simulink model "singlePhaseMMCfaultSimplev4"  (R2023b)
settings: Solver=FixedStepDiscrete  StartTime=0.0  StopTime=20  RelTol=1e-3
PreLoadFcn:
  | % Nominal system frequency (Hz)
  |     Fnom= 50;
  | % Number of power module per half-arm
  |     Nb_PM=4;
  | % Nominal DC voltage of one module (V)
  |     Vnom_PM=1000;
  | % Nominal voltage plus DC source
  |     VDCp= (Nb_PM*Vnom_PM)/2;
  | % Nominal voltage minus DC source
  |     VDCm= VDCp;
  | % Power module capacitor (F)
  |     C_PM= 1e9;
  | % Initial capacitor DC voltage (V)
  |     Vc_Initial=Vnom_PM;
  | % SPS Simulation time step(s)
  |     Ts_Power= 10e-6;
  | 
  | % Modulator Parameters:
  | % Carriers frequency (Hz)
  |     Fc=Fnom*3;
  | 
  | % Switches parameters:
  | Ron=1e-3;
  | Rs=1e6;
  | Cs=inf;
libraries: spsHalfBridgeMMCLib x8, spsSeriesRLCBranchLib x6, spsIdealSwitchLib x4, spsVoltageMeasurementLib x4, spsCurrentMeasurementLib x3, spsPWMGeneratorMultilevelLib x2, spsGroundLib x2, spsDCVoltageSourceLib x2, spspowerguiLib x1
settings Model: Creator=The MathWorks, Inc.  LastModifiedBy=broom
settings SolverCC: AlgebraicLoopSolver=TrustRegion
settings DataIOCC: SaveFormat=StructureWithTime  SaveOutput=off  SignalLogging=off  DSMLogging=off  SaveTime=off  ReturnWorkspaceOutputs=off
settings OptimizationCC: ExpressionDepthLimit=2147483647  LifeSpan=inf
settings DebuggingCC: UnderspecifiedInitializationDetection=Classic  MergeDetectMultiDrivingBlocksExec=none  SolverPrmCheckMsg=warning  FcnCallInpInsideContextMsg=warning  UnconnectedInputMsg=warning  UnconnectedOutputMsg=warning  UnconnectedLineMsg=warning  AllowSymbolicDim=off  StateNameClashWarn=warning  SFUnexpectedBacktrackingDiag=warning  SFNoUnconditionalDefaultTransitionDiag=warning  SFExecutionAtInitializationDiag=none  ArithmeticOperatorsInVariantConditions=warning
settings HardwareCC: ProdBitPerPointer=32  ProdBitPerSizeT=32  ProdBitPerPtrDiffT=32  ProdLargestAtomicFloat=None  ProdIntDivRoundTo=Undefined  ProdEndianess=Unspecified  ProdWordSize=32  ProdHWDeviceType=32-bit Generic
settings ModelReferenceCC: EnableRefExpFcnMdlSchedulingChecks=on  PropagateSignalLabelsOutOfModel=off
settings SFSimCC: SimUseLocalCustomCode=off  CustomCodeUndefinedFunction=UseInterfaceOnly
settings RTWCC: RTWUseLocalCustomCode=off
settings CodeAppCC: StateflowObjectComments=on
settings GRTTargetCC: TargetLangStandard=C89/C90 (ANSI)  CombineOutputUpdateFcns=off  GRTInterface=on
settings ConfigComp: CovMetricSettings=dw  CovSaveCumulativeToWorkspaceVar=on  CovSaveSingleToWorkspaceVar=on  CovExternalEMLEnable=off
settings SimscapeCC: SimscapeNormalizeSystem=off  SimscapeNominalValues={1, 'bar'; 1, 'cm^3/s'; 1, 'bar*kg/s'; 1, 'kJ/kg'; 1, 'kW'; }

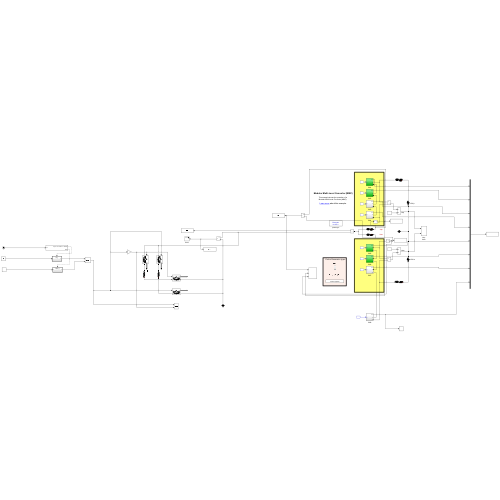
[thumbnail: Simulink's stored preview of the top-level diagram]
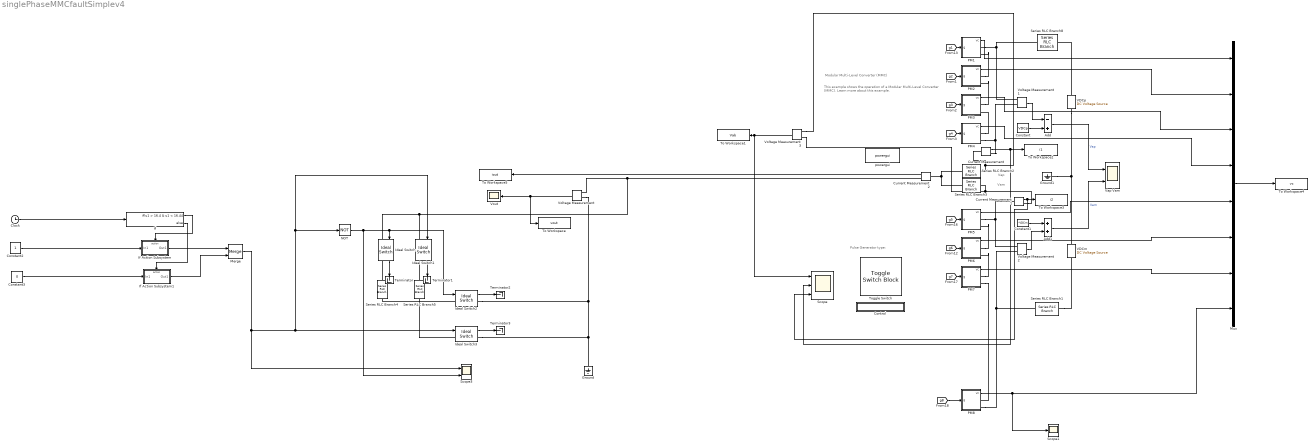
== system singlePhaseMMCfaultSimplev4 ==
  note: Pulse Generator type:
  note: Vap
  note: Vam
  note: Modular Multi-Level Converter (MMC)
  note: This example shows the operation of a
      | Modular Multi-Level Converter (MMC).
      |
      | Learn more about this example.
  Add : Sum  Inputs=-+
  Add1 : Sum
  Clock : Clock
  Constant : Constant  Value=VDCp
  Constant1 : Constant  Value=-VDCm
  Constant2 : Constant
  Constant3 : Constant  Value=0
  Control : Subsystem
      mask Display: disp('Control system')
  Current Measurement : spsCurrentMeasurementLib/Current Measurement  PhasorSimulation=off  OutputType=Complex  PSBequivalent=0
  Current Measurement1 : spsCurrentMeasurementLib/Current Measurement  PhasorSimulation=off  OutputType=Complex  PSBequivalent=0
  Current Measurement2 : spsCurrentMeasurementLib/Current Measurement  PhasorSimulation=off  OutputType=Complex  PSBequivalent=0
  Ground : spsGroundLib/Ground  LConnTagsString=a
  Ground1 : spsGroundLib/Ground  LConnTagsString=a
  Ideal Switch : spsIdealSwitchLib/Ideal Switch  Ron=0.001  Lon=0  IC=1  Rs=1e5  Cs=inf  Measurements=on
  Ideal Switch1 : spsIdealSwitchLib/Ideal Switch  Ron=0.001  Lon=0  IC=0  Rs=1e5  Cs=inf  Measurements=on
  Ideal Switch2 : spsIdealSwitchLib/Ideal Switch  Ron=0.001  Lon=0  IC=1  Rs=1e5  Cs=inf  Measurements=on
  Ideal Switch3 : spsIdealSwitchLib/Ideal Switch  Ron=0.001  Lon=0  IC=0  Rs=1e5  Cs=inf  Measurements=on
  If : If  IfExpression=u1 > 16.4 & u1 < 16.44
  If Action Subsystem : Subsystem  TreatAsAtomicUnit=on
  If Action Subsystem1 : Subsystem  TreatAsAtomicUnit=on
  Merge : Merge
  Mux : Mux  Inputs=8
  NOT : Logic  Operator=NOT  IconShape=distinctive  AllPortsSameDT=off  OutDataTypeStr=boolean
  PM1 : Subsystem
  PM2 : Subsystem
  PM3 : Subsystem
  PM4 : Subsystem
  PM5 : Subsystem
  PM6 : Subsystem
  PM7 : Subsystem
  PM8 : Subsystem
  Scope : Scope  NumInputPorts=3
  Scope1 : Scope
  Scope3 : Scope  NumInputPorts=2
  Series RLC Branch1 : spsSeriesRLCBranchLib/Series RLC Branch  LConnTagsString=__new0  RConnTagsString=__new0  BranchType=RL  Resistance=0.1  Inductance=1e-3  SetiL0=off  InitialCurrent=0  Capacitance=1e-6  Setx0=off  InitialVoltage=0  Measurements=None
  Series RLC Branch2 : spsSeriesRLCBranchLib/Series RLC Branch  LConnTagsString=__new0  RConnTagsString=__new0  BranchType=RL  Resistance=1  Inductance=10e-3  SetiL0=off  InitialCurrent=0  Capacitance=1e-6  Setx0=off  InitialVoltage=0  Measurements=None
  Series RLC Branch3 : spsSeriesRLCBranchLib/Series RLC Branch  LConnTagsString=__new0  RConnTagsString=__new0  BranchType=RL  Resistance=1  Inductance=10e-3  SetiL0=off  InitialCurrent=0  Capacitance=1e-6  Setx0=off  InitialVoltage=0  Measurements=None
  Series RLC Branch4 : spsSeriesRLCBranchLib/Series RLC Branch  LConnTagsString=__new0  RConnTagsString=__new0  BranchType=R  Resistance=50  Inductance=10e-3  SetiL0=off  InitialCurrent=0  Capacitance=1e-6  Setx0=off  InitialVoltage=0  Measurements=None
  Series RLC Branch5 : spsSeriesRLCBranchLib/Series RLC Branch  LConnTagsString=__new0  RConnTagsString=__new0  BranchType=R  Resistance=1e-9  Inductance=10e-3  SetiL0=off  InitialCurrent=0  Capacitance=1e-6  Setx0=off  InitialVoltage=0  Measurements=None
  Series RLC Branch8 : spsSeriesRLCBranchLib/Series RLC Branch  LConnTagsString=__new0  RConnTagsString=__new0  BranchType=RL  Resistance=0.1  Inductance=1e-3  SetiL0=off  InitialCurrent=0  Capacitance=1e-6  Setx0=off  InitialVoltage=0  Measurements=None
  Terminator{,1..3} (4 alike) : Terminator
  To Workspace : ToWorkspace  VariableName=vout  SaveFormat=Timeseries  SampleTime=-1
  To Workspace1 : ToWorkspace  VariableName=Vab  SaveFormat=Timeseries  SampleTime=-1
  To Workspace2 : ToWorkspace  VariableName=i1  SaveFormat=Timeseries  SampleTime=-1
  To Workspace3 : ToWorkspace  VariableName=i2  SaveFormat=Timeseries  SampleTime=-1
  To Workspace4 : ToWorkspace  VariableName=vc  SaveFormat=Timeseries  SampleTime=-1
      settings: Save2DSignal=2-D array (concatenate along first dimension)
  To Workspace5 : ToWorkspace  VariableName=iout  SaveFormat=Timeseries  SampleTime=-1
  Toggle Switch : ToggleSwitchBlock  LabelPosition=Hide
      settings: Values={{'Nearest level', 'PWM'}, [0 1]}
  VDCm : spsDCVoltageSourceLib/DC Voltage Source  Amplitude=VDCm  Measurements=None
  VDCp : spsDCVoltageSourceLib/DC Voltage Source  Amplitude=VDCp  Measurements=None
  Vap Vam : Scope  NumInputPorts=2
  Voltage Measurement{,1..3} (4 alike) : spsVoltageMeasurementLib/Voltage Measurement  PhasorSimulation=off  OutputType=Complex  PSBequivalent=0
  Vout : Scope
  powergui : spspowerguiLib/powergui  Priority=1  SimulationMode=Discrete  SampleTime=Ts_Power  frequency=60  Iterations=50  frequencyindice=0  Pbase=100e6  ErrMax=1e-4  UnitsV=kV  UnitsW=MW  buscounter=0  FunctionMessages=off  echomessages=off  EnableUseOfTLC=off  CurrentSourceSwitches=off  DisableSnubberDevices=off  DisableRonSwitches=off  DisableVfSwitches=off  DisplayEquations=off  AutomaticDiscreteSolvers=off  SolverType=Tustin/Backward Euler (TBE)  Interpol=off  ExternalGateDelay=off  methode=off  Ts=10  x0status=blocks  SPID=off  SwTol=0  HookPort=off  NonlinearTolerance=1e-4  nMaxIteration=100  ContinueOnMaxIteration=off  RestoreLinks=warning  ResistiveCurrentMeasurement=off  Frange=[0:2:500]  Ylog=off  Xlog=on  ShowGrid=off  save=off  variable=ZData  structure=Vout  ZoomFFT=on  StartTime=0.15  cycles=2  DisplayStyle=1  fundamental=50  FreqAxis=on  MaxFrequency=6000  frequencyindicesteady=1  RmsSteady=1  display=off
  wires:
  [g1] -> PM1/1(g)
  [g2] -> PM2/1(g)
  [g3] -> PM3/1(g)
  [g4] -> PM4/1(g)
  [g5] -> PM5/1(g)
  [g6] -> PM6/1(g)
  [g7] -> PM7/1(g)
  Voltage Measurement/1 -> To Workspace/1, Vout/1
  Voltage Measurement1/1 -> Add/1
  Add/1 -> Vap Vam/1  "Vap"
  Add1/1 -> Vap Vam/2  "Vam"
  Constant/1 -> Add/2
  Constant1/1 -> Add1/1
  Voltage Measurement2/1 -> Add1/2
  Voltage Measurement3/1 -> Scope/1, To Workspace1/1
  Current Measurement/1 -> To Workspace2/1, Scope/2
  Current Measurement1/1 -> Scope/3, To Workspace3/1
  PM1/1(vc) -> Mux/1
  PM2/1(vc) -> Mux/2
  PM3/1(vc) -> Mux/3
  PM4/1(vc) -> Mux/4
  PM5/1(vc) -> Mux/5
  PM6/1(vc) -> Mux/6
  PM7/1(vc) -> Mux/7
  PM8/1(vc) -> Mux/8, Scope1/1
  Mux/1 -> To Workspace4/1
  Current Measurement2/1 -> To Workspace5/1
  Ideal Switch/1 -> Terminator/1
  Ideal Switch1/1 -> Terminator1/1
  Ideal Switch2/1 -> Terminator2/1
  Ideal Switch3/1 -> Terminator3/1
  Constant2/1 -> If Action Subsystem/1(In1)
  [g8] -> PM8/1(g)
  Clock/1 -> If/1
  Constant3/1 -> If Action Subsystem1/1(In1)
  If/1 -> If Action Subsystem/Action
  If Action Subsystem/1(Out1) -> Merge/1
  If/2 -> If Action Subsystem1/Action
  If Action Subsystem1/1(Out1) -> Merge/2
  Merge/1 -> Scope3/1, Ideal Switch3/1, NOT/1, Ideal Switch1/1
  NOT/1 -> Ideal Switch2/1, Ideal Switch/1, Scope3/2
  connections:
  PM3/RConn1 -- PM2/RConn2
  PM4/RConn1 -- PM3/RConn2
  PM7/RConn1 -- PM6/RConn2
  PM6/RConn1 -- PM5/RConn2
  Voltage Measurement3/LConn2 -- Current Measurement1/RConn1 -- Series RLC Branch3/LConn1
  PM1/RConn1 -- Series RLC Branch8/RConn1 -- Voltage Measurement1/LConn1
  Series RLC Branch2/RConn1 -- Current Measurement2/LConn1 -- Series RLC Branch3/RConn1
  Voltage Measurement/LConn2 -- Ideal Switch2/RConn1 -- Ideal Switch3/RConn1 -- Ground/LConn1
  VDCp/RConn1 -- Series RLC Branch8/LConn1
  Series RLC Branch1/LConn1 -- VDCm/LConn1
  VDCp/LConn1 -- Ground1/LConn1 -- VDCm/RConn1
  Voltage Measurement3/LConn1 -- Current Measurement/LConn1 -- Series RLC Branch2/LConn1
  Voltage Measurement2/LConn2 -- Series RLC Branch1/RConn1 -- PM8/RConn2
  PM2/RConn1 -- PM1/RConn2
  PM4/RConn2 -- Voltage Measurement1/LConn2 -- Current Measurement/RConn1
  PM5/RConn1 -- Current Measurement1/LConn1 -- Voltage Measurement2/LConn1
  Current Measurement2/RConn1 -- Ideal Switch1/LConn1 -- Ideal Switch/LConn1 -- Voltage Measurement/LConn1
  PM7/RConn2 -- PM8/RConn1
  Series RLC Branch5/RConn1 -- Ideal Switch1/RConn1
  Series RLC Branch4/RConn1 -- Ideal Switch/RConn1
  Ideal Switch2/LConn1 -- Series RLC Branch4/LConn1
  Series RLC Branch5/LConn1 -- Ideal Switch3/LConn1

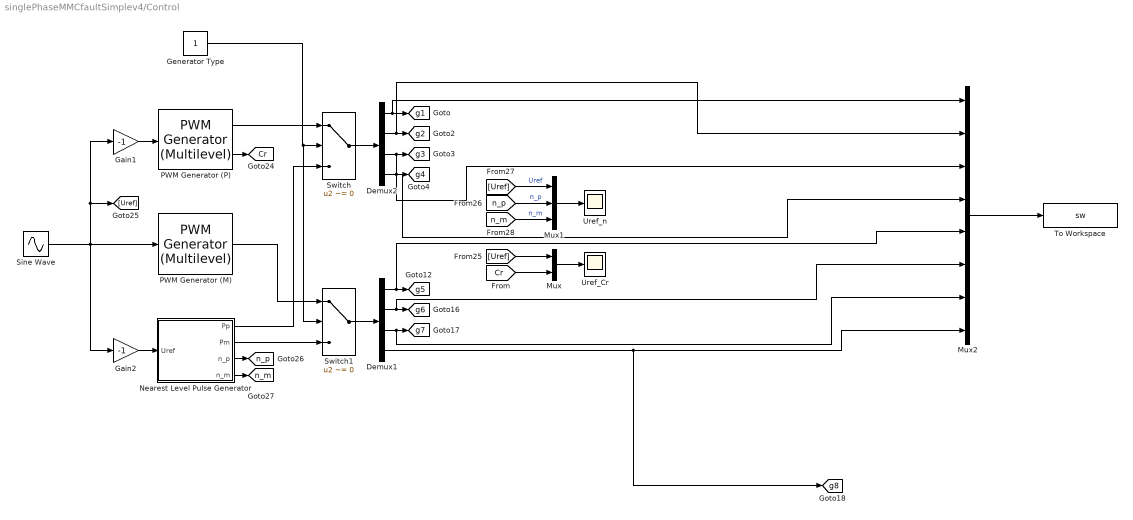
== system singlePhaseMMCfaultSimplev4/Control ==
  Demux1 : Demux  Outputs=Nb_PM
  Demux2 : Demux  Outputs=Nb_PM
  Gain1 : Gain  Gain=-1
  Gain2 : Gain  Gain=-1
  Generator Type : Constant
  Mux : Mux  Inputs=2
  Mux1 : Mux  Inputs=3
  Mux2 : Mux  Inputs=8
  "Nearest Level Pulse Generator " : Subsystem
  PWM Generator (M) : spsPWMGeneratorMultilevelLib/PWM Generator (Multilevel)  BridgeType=Half-bridge  NumberOfBridges=Nb_PM  Fc=Fc  Ts=Ts_Power  ShowCarriersOutport=off
      settings: LibrarySourceBlock=|
      | sps_lib/Power Electronics/Power Electronics Control/PWM Generator
      | (Multilevel)
  PWM Generator (P) : spsPWMGeneratorMultilevelLib/PWM Generator (Multilevel)  BridgeType=Half-bridge  NumberOfBridges=Nb_PM  Fc=Fc  Ts=Ts_Power  ShowCarriersOutport=on
      settings: LibrarySourceBlock=|
      | sps_lib/Power Electronics/Power Electronics Control/PWM Generator
      | (Multilevel)
  Sine Wave : Sin  Frequency=2*pi*50  SampleTime=Ts_Power
  Switch : Switch  Criteria=u2 ~= 0  SaturateOnIntegerOverflow=off  InputSameDT=off
  Switch1 : Switch  Criteria=u2 ~= 0  SaturateOnIntegerOverflow=off  InputSameDT=off
  To Workspace : ToWorkspace  VariableName=sw  SaveFormat=Timeseries  SampleTime=-1
  Uref_Cr : Scope
  Uref_n : Scope
  tag scope: Cr=global, g1=global, g2=global, g3=global, g4=global, g5=global, g6=global, g7=global, g8=global, n_m=global, n_p=global
  wires:
  Demux2/2 -> Mux2/2, [g2]
  Demux2/4 -> Mux2/4, [g4]
  Sine Wave/1 -> Gain1/1, [Uref], PWM Generator (M)/1, Gain2/1
  Demux1/3 -> Mux2/7, [g7]
  Switch1/1 -> Demux1/1
  Generator Type/1 -> Switch1/2, Switch/2
  Demux1/2 -> Mux2/6, [g6]
  "Nearest Level Pulse Generator "/1(Pp) -> Switch/3
  PWM Generator (P)/1 -> Switch/1
  Switch/1 -> Demux2/1
  Gain1/1 -> PWM Generator (P)/1
  "Nearest Level Pulse Generator "/2(Pm) -> Switch1/3
  Gain2/1 -> "Nearest Level Pulse Generator "/1(Uref)
  Demux2/1 -> Mux2/1, [g1]
  PWM Generator (P)/2 -> [Cr]
  Demux1/1 -> Mux2/5, [g5]
  Demux2/3 -> Mux2/3, [g3]
  PWM Generator (M)/1 -> Switch1/1
  "Nearest Level Pulse Generator "/3(n_p) -> [n_p]
  "Nearest Level Pulse Generator "/4(n_m) -> [n_m]
  Mux/1 -> Uref_Cr/1
  [Cr] -> Mux/2
  [Uref] -> Mux/1
  Mux1/1 -> Uref_n/1
  [n_p] -> Mux1/2  "n_p"
  [Uref] -> Mux1/1  "Uref"
  [n_m] -> Mux1/3  "n_m"
  Mux2/1 -> To Workspace/1
  Demux1/4 -> [g8], Mux2/8

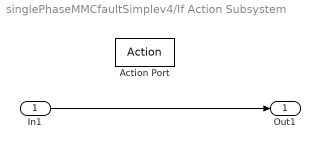
== system singlePhaseMMCfaultSimplev4/If Action Subsystem ==
  In1 : Inport
  Action Port : ActionPort  ActionPortLabel=if(u1 > 16.4 & u1 < 16.44)
  Out1 : Outport
  wires:
  In1/1 -> Out1/1

== system singlePhaseMMCfaultSimplev4/If Action Subsystem1 ==
  In1 : Inport
  Action Port : ActionPort  ActionPortLabel=else
  Out1 : Outport
  wires:
  In1/1 -> Out1/1

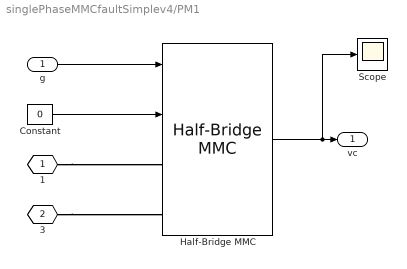
== system singlePhaseMMCfaultSimplev4/PM1 ==
  g : Inport  PortDimensions=2
  Constant : Constant  Value=0
  Half-Bridge MMC : spsHalfBridgeMMCLib/Half-Bridge MMC  ModelType=Switching devices  n=1  C=C_PM  Vc_Initial=Vc_Initial  Ron=Ron  Rs=Rs  Cs=Cs  Ron_Diode=1e-3  Rs_Diode=1e6  Cs_Diode=inf  Vf_Diode=1e-3  Rs_CurrentSource=inf  Ts=10e-6
      settings: LibrarySourceBlock=sps_lib/Power Electronics/Half-Bridge MMC
  Scope : Scope
  1 : PMIOPort  Tag=PMCPort  Side=Right
  3 : PMIOPort  Tag=PMCPort  Port=2  Side=Right
  vc : Outport
  wires:
  Constant/1 -> Half-Bridge MMC/2
  Half-Bridge MMC/1 -> Scope/1, vc/1
  g/1 -> Half-Bridge MMC/1
  connections:
  1/RConn1 -- Half-Bridge MMC/LConn1
  3/RConn1 -- Half-Bridge MMC/LConn2

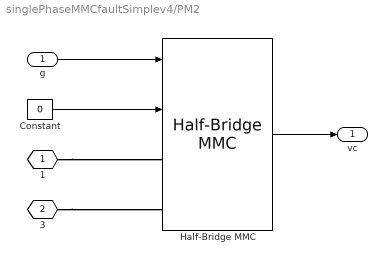
== system singlePhaseMMCfaultSimplev4/PM2 ==
  g : Inport  PortDimensions=2
  Constant : Constant  Value=0
  Half-Bridge MMC : spsHalfBridgeMMCLib/Half-Bridge MMC  ModelType=Switching devices  n=1  C=C_PM  Vc_Initial=Vc_Initial  Ron=Ron  Rs=Rs  Cs=Cs  Ron_Diode=1e-3  Rs_Diode=1e6  Cs_Diode=inf  Vf_Diode=1e-3  Rs_CurrentSource=inf  Ts=10e-6
      settings: LibrarySourceBlock=sps_lib/Power Electronics/Half-Bridge MMC
  1 : PMIOPort  Tag=PMCPort  Side=Right
  3 : PMIOPort  Tag=PMCPort  Port=2  Side=Right
  vc : Outport
  wires:
  g/1 -> Half-Bridge MMC/1
  Half-Bridge MMC/1 -> vc/1
  Constant/1 -> Half-Bridge MMC/2
  connections:
  3/RConn1 -- Half-Bridge MMC/LConn2
  1/RConn1 -- Half-Bridge MMC/LConn1

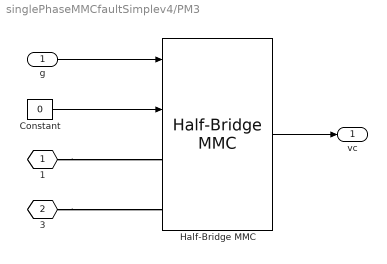
== system singlePhaseMMCfaultSimplev4/PM3 ==
  g : Inport  PortDimensions=2
  Constant : Constant  Value=0
  Half-Bridge MMC : spsHalfBridgeMMCLib/Half-Bridge MMC  ModelType=Switching devices  n=1  C=C_PM  Vc_Initial=Vc_Initial  Ron=Ron  Rs=Rs  Cs=Cs  Ron_Diode=1e-3  Rs_Diode=1e6  Cs_Diode=inf  Vf_Diode=1e-3  Rs_CurrentSource=inf  Ts=10e-6
      settings: LibrarySourceBlock=sps_lib/Power Electronics/Half-Bridge MMC
  1 : PMIOPort  Tag=PMCPort  Side=Right
  3 : PMIOPort  Tag=PMCPort  Port=2  Side=Right
  vc : Outport
  wires:
  Constant/1 -> Half-Bridge MMC/2
  Half-Bridge MMC/1 -> vc/1
  g/1 -> Half-Bridge MMC/1
  connections:
  1/RConn1 -- Half-Bridge MMC/LConn1
  3/RConn1 -- Half-Bridge MMC/LConn2

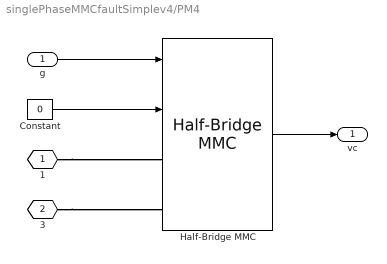
== system singlePhaseMMCfaultSimplev4/PM4 ==
  g : Inport  PortDimensions=2
  Constant : Constant  Value=0
  Half-Bridge MMC : spsHalfBridgeMMCLib/Half-Bridge MMC  ModelType=Switching devices  n=1  C=C_PM  Vc_Initial=Vc_Initial  Ron=Ron  Rs=Rs  Cs=Cs  Ron_Diode=1e-3  Rs_Diode=1e6  Cs_Diode=inf  Vf_Diode=1e-3  Rs_CurrentSource=inf  Ts=10e-6
      settings: LibrarySourceBlock=sps_lib/Power Electronics/Half-Bridge MMC
  1 : PMIOPort  Tag=PMCPort  Side=Right
  3 : PMIOPort  Tag=PMCPort  Port=2  Side=Right
  vc : Outport
  wires:
  g/1 -> Half-Bridge MMC/1
  Half-Bridge MMC/1 -> vc/1
  Constant/1 -> Half-Bridge MMC/2
  connections:
  3/RConn1 -- Half-Bridge MMC/LConn2
  1/RConn1 -- Half-Bridge MMC/LConn1

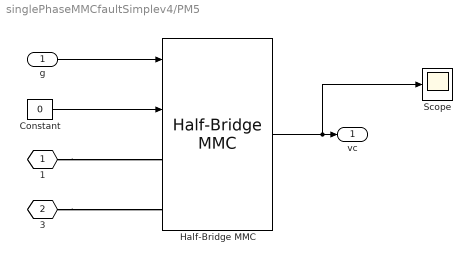
== system singlePhaseMMCfaultSimplev4/PM5 ==
  g : Inport  PortDimensions=2
  Constant : Constant  Value=0
  Half-Bridge MMC : spsHalfBridgeMMCLib/Half-Bridge MMC  ModelType=Switching devices  n=1  C=C_PM  Vc_Initial=Vc_Initial  Ron=Ron  Rs=Rs  Cs=Cs  Ron_Diode=1e-3  Rs_Diode=1e6  Cs_Diode=inf  Vf_Diode=1e-3  Rs_CurrentSource=inf  Ts=10e-6
      settings: LibrarySourceBlock=sps_lib/Power Electronics/Half-Bridge MMC
  Scope : Scope
  1 : PMIOPort  Tag=PMCPort  Side=Right
  3 : PMIOPort  Tag=PMCPort  Port=2  Side=Right
  vc : Outport
  wires:
  Constant/1 -> Half-Bridge MMC/2
  Half-Bridge MMC/1 -> Scope/1, vc/1
  g/1 -> Half-Bridge MMC/1
  connections:
  1/RConn1 -- Half-Bridge MMC/LConn1
  3/RConn1 -- Half-Bridge MMC/LConn2

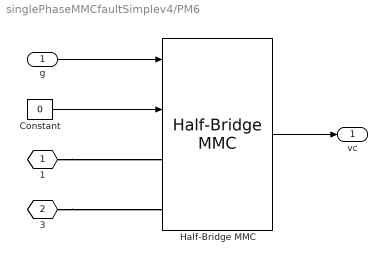
== system singlePhaseMMCfaultSimplev4/PM6 ==
  g : Inport  PortDimensions=2
  Constant : Constant  Value=0
  Half-Bridge MMC : spsHalfBridgeMMCLib/Half-Bridge MMC  ModelType=Switching devices  n=1  C=C_PM  Vc_Initial=Vc_Initial  Ron=Ron  Rs=Rs  Cs=Cs  Ron_Diode=1e-3  Rs_Diode=1e6  Cs_Diode=inf  Vf_Diode=1e-3  Rs_CurrentSource=inf  Ts=10e-6
      settings: LibrarySourceBlock=sps_lib/Power Electronics/Half-Bridge MMC
  1 : PMIOPort  Tag=PMCPort  Side=Right
  3 : PMIOPort  Tag=PMCPort  Port=2  Side=Right
  vc : Outport
  wires:
  g/1 -> Half-Bridge MMC/1
  Half-Bridge MMC/1 -> vc/1
  Constant/1 -> Half-Bridge MMC/2
  connections:
  3/RConn1 -- Half-Bridge MMC/LConn2
  1/RConn1 -- Half-Bridge MMC/LConn1

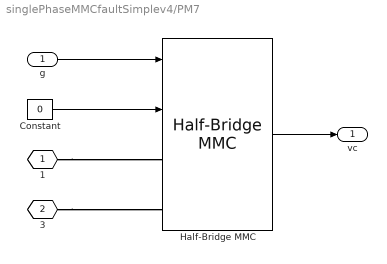
== system singlePhaseMMCfaultSimplev4/PM7 ==
  g : Inport  PortDimensions=2
  Constant : Constant  Value=0
  Half-Bridge MMC : spsHalfBridgeMMCLib/Half-Bridge MMC  ModelType=Switching devices  n=1  C=C_PM  Vc_Initial=Vc_Initial  Ron=Ron  Rs=Rs  Cs=Cs  Ron_Diode=1e-3  Rs_Diode=1e6  Cs_Diode=inf  Vf_Diode=1e-3  Rs_CurrentSource=inf  Ts=10e-6
      settings: LibrarySourceBlock=sps_lib/Power Electronics/Half-Bridge MMC
  1 : PMIOPort  Tag=PMCPort  Side=Right
  3 : PMIOPort  Tag=PMCPort  Port=2  Side=Right
  vc : Outport
  wires:
  Constant/1 -> Half-Bridge MMC/2
  Half-Bridge MMC/1 -> vc/1
  g/1 -> Half-Bridge MMC/1
  connections:
  1/RConn1 -- Half-Bridge MMC/LConn1
  3/RConn1 -- Half-Bridge MMC/LConn2

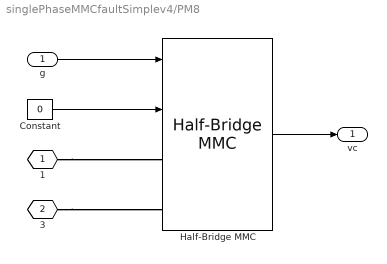
== system singlePhaseMMCfaultSimplev4/PM8 ==
  g : Inport  PortDimensions=2
  Constant : Constant  Value=0
  Half-Bridge MMC : spsHalfBridgeMMCLib/Half-Bridge MMC  ModelType=Switching devices  n=1  C=C_PM  Vc_Initial=Vc_Initial  Ron=Ron  Rs=Rs  Cs=Cs  Ron_Diode=1e-3  Rs_Diode=1e6  Cs_Diode=inf  Vf_Diode=1e-3  Rs_CurrentSource=inf  Ts=10e-6
      settings: LibrarySourceBlock=sps_lib/Power Electronics/Half-Bridge MMC
  1 : PMIOPort  Tag=PMCPort  Side=Right
  3 : PMIOPort  Tag=PMCPort  Port=2  Side=Right
  vc : Outport
  wires:
  g/1 -> Half-Bridge MMC/1
  Half-Bridge MMC/1 -> vc/1
  Constant/1 -> Half-Bridge MMC/2
  connections:
  3/RConn1 -- Half-Bridge MMC/LConn2
  1/RConn1 -- Half-Bridge MMC/LConn1

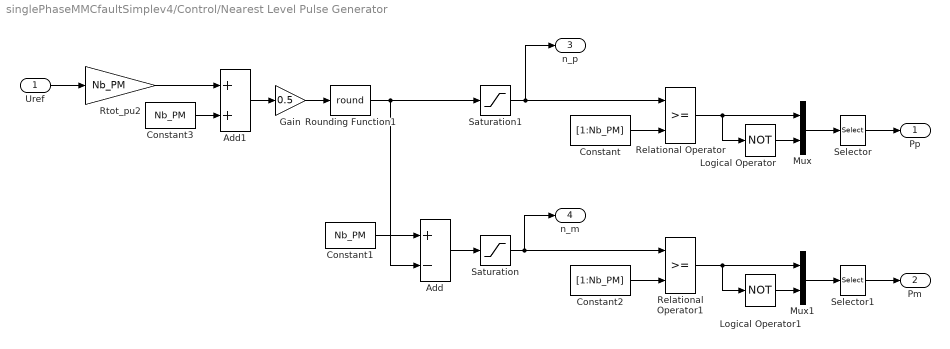
== system singlePhaseMMCfaultSimplev4/Control/Nearest Level Pulse Generator  ==
  Uref : Inport
  Add : Sum  Inputs=+-
  Add1 : Sum
  Constant : Constant  Value=[1:Nb_PM]
  Constant1 : Constant  Value=Nb_PM
  Constant2 : Constant  Value=[1:Nb_PM]
  Constant3 : Constant  Value=Nb_PM
  Gain : Gain  Gain=0.5
  Logical Operator : Logic  Operator=NOT  AllPortsSameDT=off  OutDataTypeStr=float('double')
  Logical Operator1 : Logic  Operator=NOT  AllPortsSameDT=off  OutDataTypeStr=float('double')
  Mux : Mux  Inputs=2
  Mux1 : Mux  Inputs=2
  Relational Operator : RelationalOperator  OutDataTypeStr=float('double')  InputSameDT=off
  Relational Operator1 : RelationalOperator  OutDataTypeStr=float('double')  InputSameDT=off
  Rounding Function1 : Rounding  Operator=round
  Rtot_pu2 : Gain  Gain=Nb_PM  SaturateOnIntegerOverflow=on  OutDataTypeStr=Inherit: Same as input  ParamDataTypeStr=Inherit: Same as input
  Saturation : Saturate  UpperLimit=Nb_PM  LowerLimit=0
  Saturation1 : Saturate  UpperLimit=Nb_PM  LowerLimit=0
  Selector : Selector  InputPortWidth=Nb_PM*2  IndexOptions=Index vector (dialog)  Indices=[1 5 2 6 3 7 4 8]  OutputSizes=1
  Selector1 : Selector  InputPortWidth=Nb_PM*2  IndexOptions=Index vector (dialog)  Indices=[1 5 2 6 3 7 4 8]  OutputSizes=1
  Pp : Outport  VectorParamsAs1DForOutWhenUnconnected=off
  Pm : Outport  Port=2  VectorParamsAs1DForOutWhenUnconnected=off
  n_p : Outport  Port=3  VectorParamsAs1DForOutWhenUnconnected=off
  n_m : Outport  Port=4  VectorParamsAs1DForOutWhenUnconnected=off
  wires:
  Constant/1 -> Relational Operator/2
  Relational Operator/1 -> Logical Operator/1, Mux/1
  Logical Operator/1 -> Mux/2
  Mux/1 -> Selector/1
  Selector/1 -> Pp/1
  Add/1 -> Saturation/1
  Constant1/1 -> Add/1
  Saturation1/1 -> n_p/1, Relational Operator/1
  Rtot_pu2/1 -> Add1/1
  Constant3/1 -> Add1/2
  Add1/1 -> Gain/1
  Gain/1 -> Rounding Function1/1
  Rounding Function1/1 -> Add/2, Saturation1/1
  Uref/1 -> Rtot_pu2/1
  Constant2/1 -> Relational Operator1/2
  Relational Operator1/1 -> Mux1/1, Logical Operator1/1
  Logical Operator1/1 -> Mux1/2
  Mux1/1 -> Selector1/1
  Selector1/1 -> Pm/1
  Saturation/1 -> n_m/1, Relational Operator1/1
